simulink model "model_matlab"  (R2022a)
settings: Solver=VariableStepAuto  StartTime=0.0  StopTime=10  RelTol=1e-3
values from neighbouring files (symbols this model uses):
  B = 1e-08    [parameter.mat]    (also in parameter_2.mat = 7.88489e-05)
  g = 9.81    [parameter.mat]    (also in parameter_2.mat = 9.8)
  J = 0.001    [parameter.mat]    (also in parameter_2.mat = 5.3e-07)
  k = 0.4    [parameter_2.mat]
  Kb = 1.9099e-07    [parameter.mat]    (also in parameter_2.mat = 0.00767)
  Km = 0.0006876    [parameter.mat]    (also in parameter_2.mat = 0.00767)
  L = 1.2e-05    [parameter.mat]    (also in parameter_2.mat = 0.00018)
  R = 3.9    [parameter.mat]    (also in parameter_2.mat = 2.6)
libraries: slpidlib x2
settings Model: Creator=ngovi  LastModifiedBy=ngovi

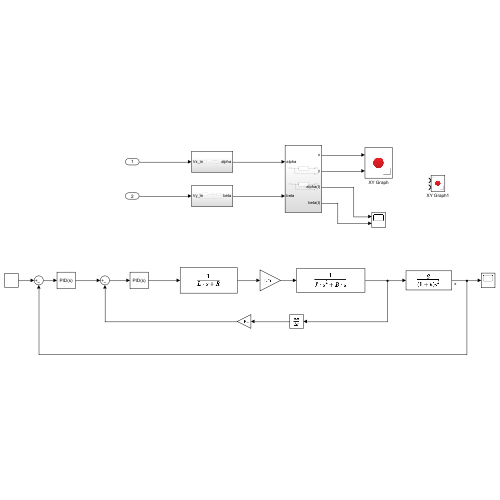
[thumbnail: Simulink's stored preview of the top-level diagram]
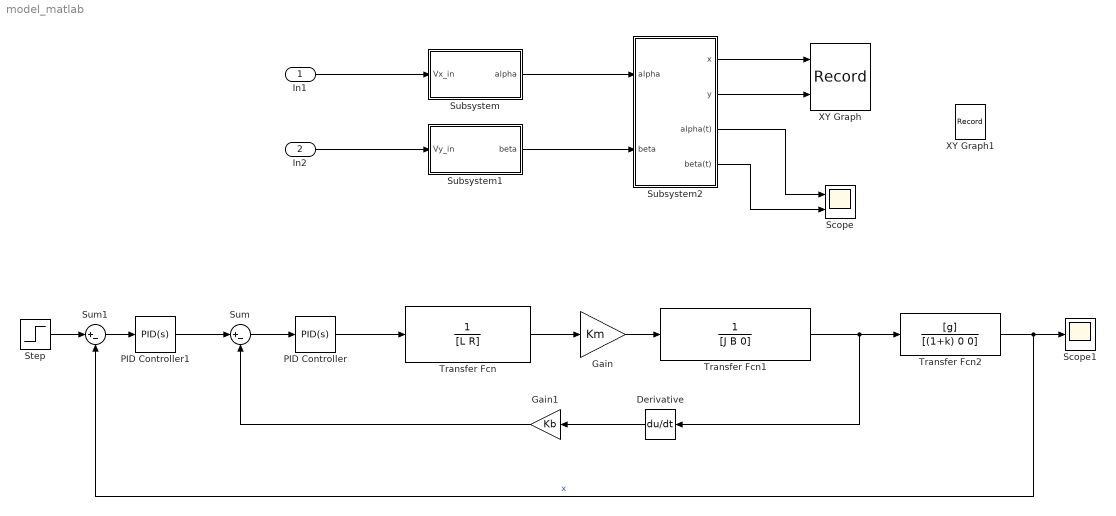
== system model_matlab ==
  In1 : Inport
  In2 : Inport  Port=2
  Derivative : Derivative
  Gain : Gain  Gain=Km
  Gain1 : Gain  Gain=Kb
  PID Controller : slpidlib/PID Controller  Controller=PID  Form=Parallel  TimeDomain=Continuous-time  UseExternalTs=off  SampleTime=-1  IntegratorMethod=Forward Euler  FilterMethod=Forward Euler  ControllerParametersSource=internal  P=0.3  I=0  UseKiTs=off  D=0.01  N=100  UseFilter=on  TunerSelectOption=Transfer Function Based (PID Tuner App)  InitialConditionSource=internal  InitialConditionForIntegrator=0  InitialConditionForFilter=0  DifferentiatorICPrevScaledInput=0  ExternalReset=none  TrackingMode=off  Kt=1  LimitOutput=off  SatLimitsSource=internal  UpperSaturationLimit=inf  LowerSaturationLimit=-inf  LinearizeAsGain=on  AntiWindupMode=none  Kb=1  POutMin=[]  POutMax=[]  IOutMin=[]  IOutMax=[]  DOutMin=[]  DOutMax=[]  NOutMin=[]  NOutMax=[]  SumOutMin=[]  SumOutMax=[]  SaturationOutMin=[]  SaturationOutMax=[]  PParamMin=[]  PParamMax=[]  IParamMin=[]  IParamMax=[]  DParamMin=[]  DParamMax=[]  NParamMin=[]  NParamMax=[]  KbParamMin=[]  KbParamMax=[]  KtParamMin=[]  KtParamMax=[]  KbOutMin=[]  KbOutMax=[]  KtOutMin=[]  KtOutMax=[]  IntegratorOutMin=[]  IntegratorOutMax=[]  FilterOutMin=[]  FilterOutMax=[]  SumI1OutMin=[]  SumI1OutMax=[]  SumI2OutMin=[]  SumI2OutMax=[]  SumI3OutMin=[]  SumI3OutMax=[]  SumI4OutMin=[]  SumI4OutMax=[]  SumDOutMin=[]  SumDOutMax=[]  DifferentiatorOutMin=[]  DifferentiatorOutMax=[]  FilterDiffOutCoefMin=[]  FilterDiffOutCoefMax=[]  ReciprocalOutMin=[]  ReciprocalOutMax=[]  SumDenOutMin=[]  SumDenOutMax=[]  SumNumOutMin=[]  SumNumOutMax=[]  DivideOutMin=[]  DivideOutMax=[]  UdiffTsProdOutMin=[]  UdiffTsProdOutMax=[]  NTsProdOutMin=[]  NTsProdOutMax=[]  UintegralTsProdOutMin=[]  UintegralTsProdOutMax=[]  UngainTsProdOutMin=[]  UngainTsProdOutMax=[]  IntegratorContinuousStateAttributes=''  IntegratorStateMustResolveToSignalObject=off  IntegratorRTWStateStorageClass=Auto  FilterContinuousStateAttributes=''  FilterStateMustResolveToSignalObject=off  FilterRTWStateStorageClass=Auto  ParallelPVariant=InternalParameters  IdealPVariant=Disabled  IVariant=InternalParameters  DVariant=InternalParameters  IntegratorVariant=Continuous  SatVariant=Disabled  AWVariant=Passthrough  PCopyVariant=Disabled  TRVariant=Disabled  FdbkBlocksVariant=Forward  IdealPFdbkVariant=Disabled  SatFdbkVariant=Disabled  DerivativeFilterVariant=ContFilter  NVariant=InternalParameters  NCopyVariant=Disabled  FilterICVariant=InternalICsFilter  IntegratorICVariant=InternalICs  ExternalResetVariant=Disabled  TRSumVariant=Passthrough  SumFdbkVariant=Disabled  SumVariant=Sum_PID  TsampFilterVariant=InternalTs  TsampNgainVariant=Passthrough  TsampIntegralVariant=Passthrough  ExternalSaturationOutDataTypeStr=Inherit: Same as second input  aMode=0
  PID Controller1 : slpidlib/PID Controller  Controller=PID  Form=Parallel  TimeDomain=Continuous-time  UseExternalTs=off  SampleTime=-1  IntegratorMethod=Forward Euler  FilterMethod=Forward Euler  ControllerParametersSource=internal  P=0.1  I=0.005  UseKiTs=off  D=1  N=100  UseFilter=on  TunerSelectOption=Transfer Function Based (PID Tuner App)  InitialConditionSource=internal  InitialConditionForIntegrator=0  InitialConditionForFilter=0  DifferentiatorICPrevScaledInput=0  ExternalReset=none  TrackingMode=off  Kt=1  LimitOutput=off  SatLimitsSource=internal  UpperSaturationLimit=inf  LowerSaturationLimit=-inf  LinearizeAsGain=on  AntiWindupMode=none  Kb=1  POutMin=[]  POutMax=[]  IOutMin=[]  IOutMax=[]  DOutMin=[]  DOutMax=[]  NOutMin=[]  NOutMax=[]  SumOutMin=[]  SumOutMax=[]  SaturationOutMin=[]  SaturationOutMax=[]  PParamMin=[]  PParamMax=[]  IParamMin=[]  IParamMax=[]  DParamMin=[]  DParamMax=[]  NParamMin=[]  NParamMax=[]  KbParamMin=[]  KbParamMax=[]  KtParamMin=[]  KtParamMax=[]  KbOutMin=[]  KbOutMax=[]  KtOutMin=[]  KtOutMax=[]  IntegratorOutMin=[]  IntegratorOutMax=[]  FilterOutMin=[]  FilterOutMax=[]  SumI1OutMin=[]  SumI1OutMax=[]  SumI2OutMin=[]  SumI2OutMax=[]  SumI3OutMin=[]  SumI3OutMax=[]  SumI4OutMin=[]  SumI4OutMax=[]  SumDOutMin=[]  SumDOutMax=[]  DifferentiatorOutMin=[]  DifferentiatorOutMax=[]  FilterDiffOutCoefMin=[]  FilterDiffOutCoefMax=[]  ReciprocalOutMin=[]  ReciprocalOutMax=[]  SumDenOutMin=[]  SumDenOutMax=[]  SumNumOutMin=[]  SumNumOutMax=[]  DivideOutMin=[]  DivideOutMax=[]  UdiffTsProdOutMin=[]  UdiffTsProdOutMax=[]  NTsProdOutMin=[]  NTsProdOutMax=[]  UintegralTsProdOutMin=[]  UintegralTsProdOutMax=[]  UngainTsProdOutMin=[]  UngainTsProdOutMax=[]  IntegratorContinuousStateAttributes=''  IntegratorStateMustResolveToSignalObject=off  IntegratorRTWStateStorageClass=Auto  FilterContinuousStateAttributes=''  FilterStateMustResolveToSignalObject=off  FilterRTWStateStorageClass=Auto  ParallelPVariant=InternalParameters  IdealPVariant=Disabled  IVariant=InternalParameters  DVariant=InternalParameters  IntegratorVariant=Continuous  SatVariant=Disabled  AWVariant=Passthrough  PCopyVariant=Disabled  TRVariant=Disabled  FdbkBlocksVariant=Forward  IdealPFdbkVariant=Disabled  SatFdbkVariant=Disabled  DerivativeFilterVariant=ContFilter  NVariant=InternalParameters  NCopyVariant=Disabled  FilterICVariant=InternalICsFilter  IntegratorICVariant=InternalICs  ExternalResetVariant=Disabled  TRSumVariant=Passthrough  SumFdbkVariant=Disabled  SumVariant=Sum_PID  TsampFilterVariant=InternalTs  TsampNgainVariant=Passthrough  TsampIntegralVariant=Passthrough  ExternalSaturationOutDataTypeStr=Inherit: Same as second input  aMode=0
  Scope : Scope  NumInputPorts=2
  Scope1 : Scope
  Step : Step  Time=0  SampleTime=0
  Subsystem : Subsystem
  Subsystem1 : Subsystem
  Subsystem2 : Subsystem
  Sum : Sum  Inputs=|+-
  Sum1 : Sum  Inputs=|+-
  Transfer Fcn : TransferFcn  Denominator=[L R]
  Transfer Fcn1 : TransferFcn  Denominator=[J B 0]
  Transfer Fcn2 : TransferFcn  Numerator=[g]  Denominator=[(1+k) 0 0]
  XY Graph : Record  FileSettingsInternal="{\"entries\":[{\"content\":{\"excelSettings\":{\"content\":{},\"type\":\"Streamout.ExcelSettings\"}},\"type\":\"Streamout.FileSettingStorage\",\"uuid\":\"78a4e250-05e6-44e0-a78a-87220abd5dd2\"}],\"packageUris\":[\"http://schema.mathworks.com/mf0/streamout_blocks/R2020a\"],\"version\":\"1.0\"}"  Layout=[1 1]  SignalsInternal="{\"entries\":[{\"content\":{\"signals\":[{\"content\":{\"blockPath\":[\"model_matlab/XY Graph\"],\"channel\":[],\"dimensions\":[1],\"domain\":\"model_matlab/XY Graph\",\"lineColor\":\"#a2142f\",\"plots\":[1],\"port\":1,\"sid\":[\"\"],\"signalID\":1550,\"signalName\":\"Subsystem2:1\"},\"type\":\"RecordBlkView.Signal\",\"uuid\":\"2434c325-6ec6-40bb-8e19-f466674402e7\"},{\"content\":{\"blockPath\":[\"model_matlab/XY Graph\"],\"channel\":[],\"dimensions\":[1],\"domain\":\"model_matlab/XY Graph\",\"lineColor\":\"#139fff\",\"plots\":[1],\"port\":2,\"sid\":[\"\"],\"signalID\":1554,\"signalName\":\"Subsystem2:2\"},\"type\":\"RecordBlkView.Signal\",\"uuid\":\"eedcce02-0f9c-4a43-b856-fd5ff02bbe51\"}]},\"type\":\"RecordBlkView.InputSignals\",\"uuid\":\"17586666-e351-4029-939d-e5dcc6d71caa\"}],\"packageUris\":[\"http://schema.mathworks.com/mf0/streamout_blocks/R2020a\"],\"version\":\"1.0\"}"  VisualizationBindings="{\"xyplotplugin\":{\"info\":[{\"series\":[{\"bindingParametersList\":[{\"parameter\":\"X-Axis\",\"signalID\":1550,\"signalName\":\"Subsystem2:1\"},{\"parameter\":\"Y-Axis\",\"signalID\":1554,\"signalName\":\"Subsystem2:2\"}],\"seriesID\":64349}],\"subplotID\":1}]}}"  CompatibilityTag=XY
  XY Graph1 : Record  FileSettingsInternal="{\"entries\":[{\"content\":{\"excelSettings\":{\"content\":{},\"type\":\"Streamout.ExcelSettings\"}},\"type\":\"Streamout.FileSettingStorage\",\"uuid\":\"cc699d7d-bb06-4ba3-9f45-c4fb237144e4\"}],\"packageUris\":[\"http://schema.mathworks.com/mf0/streamout_blocks/R2020a\"],\"version\":\"1.0\"}"  Layout=[1 1]  SignalsInternal="{\"entries\":[{\"content\":{\"signals\":[{\"content\":{\"blockPath\":[\"model_matlab/XY Graph1\"],\"channel\":[],\"dimensions\":[1],\"domain\":\"model_matlab/XY Graph1\",\"lineColor\":\"#a2142f\",\"plots\":[1],\"port\":1,\"sid\":[\"\"],\"signalID\":1558},\"type\":\"RecordBlkView.Signal\",\"uuid\":\"f283e571-f734-4db6-a1ed-ae672e17f0ba\"},{\"content\":{\"blockPath\":[\"model_matlab/XY Graph1\"],\"channel\":[],\"dimensions\":[1],\"domain\":\"model_matlab/XY Graph1\",\"lineColor\":\"#139fff\",\"plots\":[1],\"port\":2,\"sid\":[\"\"],\"signalID\":1562},\"type\":\"RecordBlkView.Signal\",\"uuid\":\"1e114b10-0667-4331-a31e-4110f9f42671\"}]},\"type\":\"RecordBlkView.InputSignals\",\"uuid\":\"85ce84d8-004b-4d2a-b343-a6eefeed6791\"}],\"packageUris\":[\"http://schema.mathworks.com/mf0/streamout_blocks/R2020a\"],\"version\":\"1.0\"}"  VisualizationBindings="{\"xyplotplugin\":{\"info\":[{\"series\":[{\"bindingParametersList\":[{\"parameter\":\"X-Axis\",\"signalID\":1558,\"signalName\":\"XY Graph1:1\"},{\"parameter\":\"Y-Axis\",\"signalID\":1562,\"signalName\":\"XY Graph1:2\"}],\"seriesID\":47058}],\"subplotID\":1}]}}"  CompatibilityTag=XY  st=-1
  wires:
  In1/1 -> Subsystem/1(Vx_in)
  In2/1 -> Subsystem1/1(Vy_in)
  Subsystem2/1(x) -> XY Graph/1
  Subsystem2/2(y) -> XY Graph/2
  Subsystem/1(alpha) -> Subsystem2/1(alpha)
  Subsystem1/1(beta) -> Subsystem2/2(beta)
  Subsystem2/3(alpha(t)) -> Scope/1
  Subsystem2/4(beta(t)) -> Scope/2
  Gain1/1 -> Sum/2
  Transfer Fcn1/1 -> Transfer Fcn2/1, Derivative/1
  Gain/1 -> Transfer Fcn1/1
  Transfer Fcn/1 -> Gain/1
  Sum/1 -> PID Controller/1
  PID Controller/1 -> Transfer Fcn/1
  Derivative/1 -> Gain1/1
  PID Controller1/1 -> Sum/1
  Sum1/1 -> PID Controller1/1
  Step/1 -> Sum1/1
  Transfer Fcn2/1 -> Sum1/2, Scope1/1  "x"

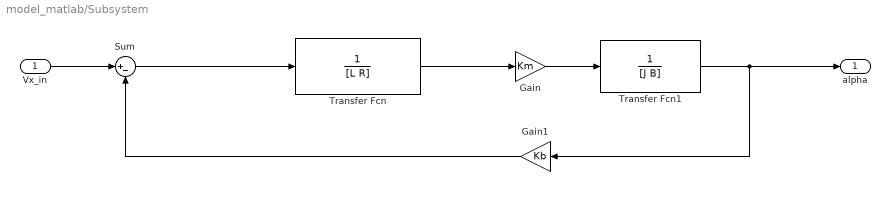
== system model_matlab/Subsystem ==
  Vx_in : Inport
  Gain : Gain  Gain=Km
  Gain1 : Gain  Gain=Kb
  Sum : Sum  Inputs=|+-
  Transfer Fcn : TransferFcn  Denominator=[L R]
  Transfer Fcn1 : TransferFcn  Denominator=[J B]
  alpha : Outport
  wires:
  Transfer Fcn/1 -> Gain/1
  Gain/1 -> Transfer Fcn1/1
  Sum/1 -> Transfer Fcn/1
  Transfer Fcn1/1 -> Gain1/1, alpha/1
  Vx_in/1 -> Sum/1
  Gain1/1 -> Sum/2

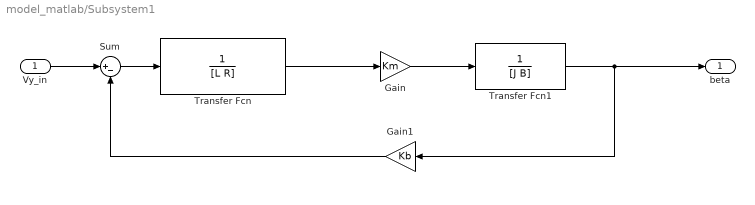
== system model_matlab/Subsystem1 ==
  Vy_in : Inport
  Gain : Gain  Gain=Km
  Gain1 : Gain  Gain=Kb
  Sum : Sum  Inputs=|+-
  Transfer Fcn : TransferFcn  Denominator=[L R]
  Transfer Fcn1 : TransferFcn  Denominator=[J B]
  beta : Outport
  wires:
  Gain1/1 -> Sum/2
  Vy_in/1 -> Sum/1
  Transfer Fcn1/1 -> Gain1/1, beta/1
  Sum/1 -> Transfer Fcn/1
  Gain/1 -> Transfer Fcn1/1
  Transfer Fcn/1 -> Gain/1

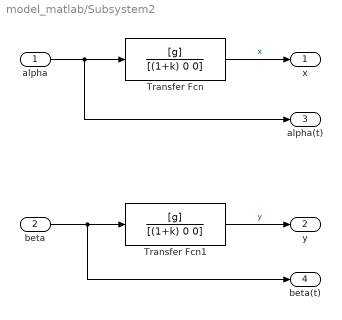
== system model_matlab/Subsystem2 ==
  alpha : Inport
  beta : Inport  Port=2
  Transfer Fcn : TransferFcn  Numerator=[g]  Denominator=[(1+k) 0 0]
  Transfer Fcn1 : TransferFcn  Numerator=[g]  Denominator=[(1+k) 0 0]
  x : Outport
  y : Outport  Port=2
  alpha(t) : Outport  Port=3
  beta(t) : Outport  Port=4
  wires:
  Transfer Fcn/1 -> x/1  "x"
  alpha/1 -> alpha(t)/1, Transfer Fcn/1
  beta/1 -> beta(t)/1, Transfer Fcn1/1
  Transfer Fcn1/1 -> y/1  "y"
